simulink model "gmStateSpaceHDL_uz_inverter_3ph"  (R2021b)
settings: Solver=FixedStepDiscrete  StartTime=0.0  StopTime=0.1  FixedStep=Auto  RelTol=1e-3
InitFcn:
  | load('C:\Users\valen\Documents\repos\2021_10_hoppe_hoerner_regelung_neunstraengige_pmsm\sschdl\uz_inverter_3ph\stateSpaceParameters.mat');
values from neighbouring files (symbols this model uses):
  udc = 200    [uz_inverter_3ph_init_parameter.m]
undefined symbols (not defined in the file or in its folder): stateSpaceParameters_1
libraries: simulink x17, hdlsllib x2, hdlssclib x2
settings Model: Creator=LENOVO  LastModifiedBy=valen
settings SolverCC: AlgebraicLoopSolver=TrustRegion
settings DataIOCC: LimitDataPoints=on  SaveOutput=off  SaveTime=off
settings OptimizationCC: BlockReduction=off  ConditionallyExecuteInputs=off  DefaultParameterBehavior=Inlined  InheritOutputTypeSmallerThanSingle=on  LifeSpan=inf
settings DebuggingCC: AlgebraicLoopMsg=error  SingleTaskRateTransMsg=error  AllowSymbolicDim=off  StrictBusMsg=ErrorOnBusTreatedAsVector  SFUnexpectedBacktrackingDiag=warning  SFNoUnconditionalDefaultTransitionDiag=warning  SFExecutionAtInitializationDiag=none  SFMachineParentedDataDiag=warning  ArithmeticOperatorsInVariantConditions=warning
settings HardwareCC: ProdBitPerPointer=32  ProdBitPerSizeT=32  ProdBitPerPtrDiffT=32  ProdLargestAtomicFloat=None  ProdIntDivRoundTo=Undefined  ProdEndianess=Unspecified  ProdWordSize=32  ProdHWDeviceType=ASIC/FPGA->ASIC/FPGA  ProdEqTarget=off
settings SFSimCC: SimUseLocalCustomCode=off  CustomCodeUndefinedFunction=UseInterfaceOnly
settings RTWCC: RTWUseLocalCustomCode=off
settings CodeAppCC: StateflowObjectComments=on
settings GRTTargetCC: TargetLangStandard=C89/C90 (ANSI)
settings ConfigComp: CovScope=ReferencedModels  CovMetricSettings=dw  CovSaveCumulativeToWorkspaceVar=on  CovSaveSingleToWorkspaceVar=on  CovExternalEMLEnable=off  CovSFcnEnable=off

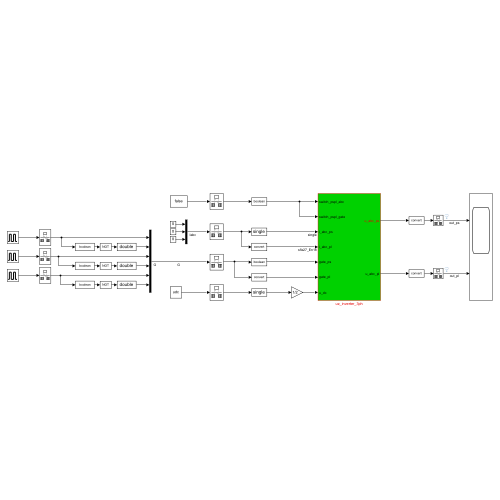
[thumbnail: Simulink's stored preview of the top-level diagram]
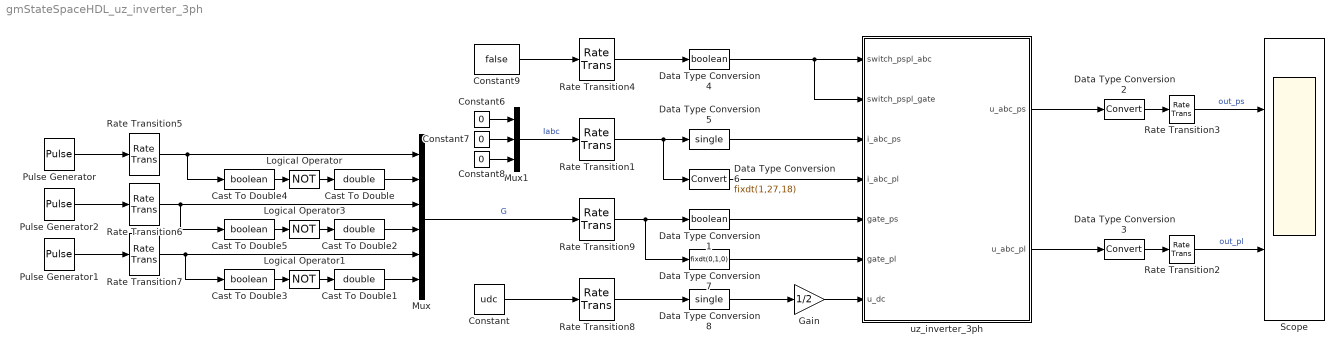
== system gmStateSpaceHDL_uz_inverter_3ph ==
  Cast To Double : DataTypeConversion  OutDataTypeStr=double
  Cast To Double1 : DataTypeConversion  OutDataTypeStr=double
  Cast To Double2 : DataTypeConversion  OutDataTypeStr=double
  Cast To Double3 : DataTypeConversion  OutDataTypeStr=boolean
  Cast To Double4 : DataTypeConversion  OutDataTypeStr=boolean
  Cast To Double5 : DataTypeConversion  OutDataTypeStr=boolean
  Constant : Constant  Value=udc
  Constant6 : Constant  Value=0
  Constant7 : Constant  Value=0
  Constant8 : Constant  Value=0
  Constant9 : Constant  Value=false
  Data Type Conversion1 : DataTypeConversion  OutDataTypeStr=boolean  RndMeth=Nearest
  Data Type Conversion2 : DataTypeConversion
  Data Type Conversion3 : DataTypeConversion
  Data Type Conversion4 : DataTypeConversion  OutDataTypeStr=boolean
  Data Type Conversion5 : DataTypeConversion  OutDataTypeStr=single  RndMeth=Nearest
  Data Type Conversion6 : DataTypeConversion  OutDataTypeStr=fixdt(1,27,18)  RndMeth=Nearest
  Data Type Conversion7 : DataTypeConversion  OutDataTypeStr=fixdt(0,1,0)  RndMeth=Nearest
  Data Type Conversion8 : DataTypeConversion  OutDataTypeStr=single  RndMeth=Nearest
  Gain : Gain  Gain=1/2  OutDataTypeStr=Inherit: Same as input
  Logical Operator : Logic  Operator=NOT  AllPortsSameDT=off  OutDataTypeStr=boolean
  Logical Operator1 : Logic  Operator=NOT  AllPortsSameDT=off  OutDataTypeStr=boolean
  Logical Operator3 : Logic  Operator=NOT  AllPortsSameDT=off  OutDataTypeStr=boolean
  Mux : Mux  Inputs=6
  Mux1 : Mux  Inputs=3
  Pulse Generator : DiscretePulseGenerator  PulseType=Time based  Period=0.001  PulseWidth=50
  Pulse Generator1 : DiscretePulseGenerator  PulseType=Time based  Period=0.01  PulseWidth=50
  Pulse Generator2 : DiscretePulseGenerator  PulseType=Time based  Period=0.05  PulseWidth=50
  Rate Transition{1..9} (9 alike) : RateTransition  OutPortSampleTime=ts_inverter
  Scope : Scope  NumInputPorts=2
  uz_inverter_3ph : Subsystem
  wires:
  uz_inverter_3ph/1(u_abc_ps) -> Data Type Conversion2/1
  uz_inverter_3ph/2(u_abc_pl) -> Data Type Conversion3/1
  Data Type Conversion3/1 -> Rate Transition2/1
  Data Type Conversion2/1 -> Rate Transition3/1
  Rate Transition3/1 -> Scope/1  "out_ps"
  Rate Transition2/1 -> Scope/2  "out_pl"
  Constant9/1 -> Rate Transition4/1
  Rate Transition4/1 -> Data Type Conversion4/1
  Mux1/1 -> Rate Transition1/1  "Iabc"
  Constant8/1 -> Mux1/3
  Constant6/1 -> Mux1/1
  Constant7/1 -> Mux1/2
  Rate Transition1/1 -> Data Type Conversion5/1, Data Type Conversion6/1
  Data Type Conversion6/1 -> uz_inverter_3ph/4(i_abc_pl)
  Rate Transition9/1 -> Data Type Conversion7/1, Data Type Conversion1/1
  Data Type Conversion1/1 -> uz_inverter_3ph/5(gate_ps)
  Data Type Conversion5/1 -> uz_inverter_3ph/3(i_abc_ps)
  Data Type Conversion7/1 -> uz_inverter_3ph/6(gate_pl)
  Logical Operator1/1 -> Cast To Double1/1
  Cast To Double3/1 -> Logical Operator1/1
  Pulse Generator1/1 -> Rate Transition7/1
  Cast To Double5/1 -> Logical Operator3/1
  Logical Operator3/1 -> Cast To Double2/1
  Pulse Generator2/1 -> Rate Transition6/1
  Pulse Generator/1 -> Rate Transition5/1
  Cast To Double2/1 -> Mux/4
  Cast To Double4/1 -> Logical Operator/1
  Cast To Double1/1 -> Mux/6
  Logical Operator/1 -> Cast To Double/1
  Mux/1 -> Rate Transition9/1  "G"
  Cast To Double/1 -> Mux/2
  Rate Transition7/1 -> Cast To Double3/1, Mux/5
  Data Type Conversion8/1 -> Gain/1
  Constant/1 -> Rate Transition8/1
  Rate Transition8/1 -> Data Type Conversion8/1
  Gain/1 -> uz_inverter_3ph/7(u_dc)
  Rate Transition6/1 -> Cast To Double5/1, Mux/3
  Rate Transition5/1 -> Cast To Double4/1, Mux/1
  Data Type Conversion4/1 -> uz_inverter_3ph/2(switch_pspl_gate), uz_inverter_3ph/1(switch_pspl_abc)

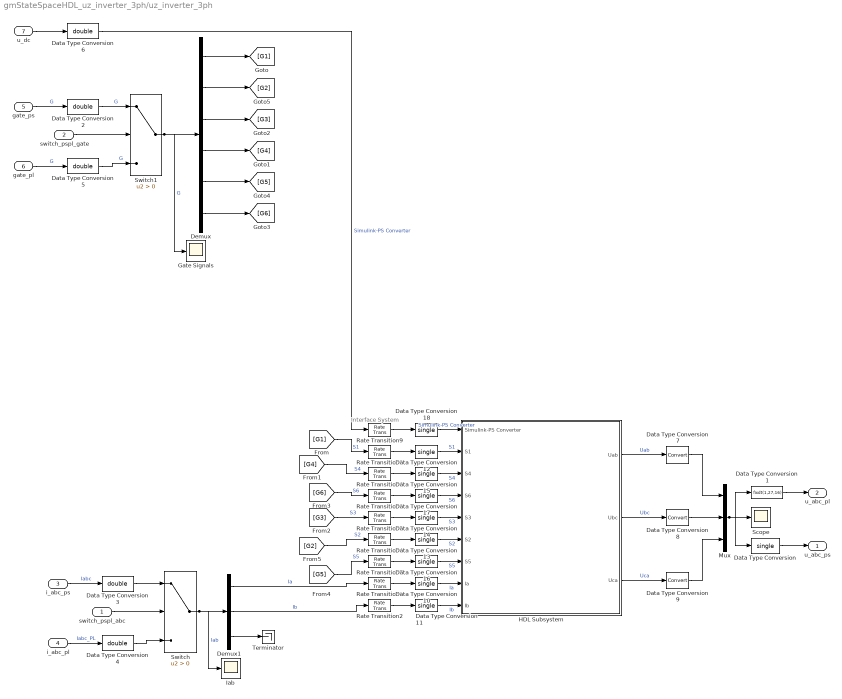
== system gmStateSpaceHDL_uz_inverter_3ph/uz_inverter_3ph ==
  note: Interface System
  switch_pspl_abc : Inport
  switch_pspl_gate : Inport  Port=2
  i_abc_ps : Inport  Port=3  OutDataTypeStr=single
  i_abc_pl : Inport  Port=4  OutDataTypeStr=fixdt(1,27,18)
  gate_ps : Inport  Port=5  LockScale=on
  gate_pl : Inport  Port=6  LockScale=on
  u_dc : Inport  Port=7
  Data Type Conversion{,10..18} (10 alike) : DataTypeConversion  OutDataTypeStr=single  RndMeth=Nearest
  Data Type Conversion1 : DataTypeConversion  OutDataTypeStr=fixdt(1,27,16)  RndMeth=Nearest
  Data Type Conversion{2..6} (5 alike) : DataTypeConversion  OutDataTypeStr=double  RndMeth=Nearest
  Data Type Conversion7 : DataTypeConversion  RndMeth=Nearest
  Data Type Conversion8 : DataTypeConversion  RndMeth=Nearest
  Data Type Conversion9 : DataTypeConversion  RndMeth=Nearest
  Demux : Demux  Outputs=6
  Demux1 : Demux  Outputs=3
  Gate Signals : Scope
  HDL Subsystem : Subsystem
  Iab : Scope
  Mux : Mux  Inputs=3
  Rate Transition{1..9} (9 alike) : RateTransition  OutPortSampleTime=1e-06
  Scope : Scope
  Switch : Switch  Criteria=u2 > Threshold
  Switch1 : Switch  Criteria=u2 > Threshold
  Terminator : Terminator
  u_abc_ps : Outport
  u_abc_pl : Outport  Port=2
  wires:
  Data Type Conversion17/1 -> HDL Subsystem/4(S6)  "S6"
  Rate Transition3/1 -> Data Type Conversion12/1
  Data Type Conversion16/1 -> HDL Subsystem/7(S5)  "S5"
  Mux/1 -> Data Type Conversion/1, Scope/1, Data Type Conversion1/1
  Rate Transition9/1 -> Data Type Conversion18/1
  Data Type Conversion10/1 -> HDL Subsystem/8(Ia)  "Ia"
  Data Type Conversion11/1 -> HDL Subsystem/9(Ib)  "Ib"
  Data Type Conversion5/1 -> Switch1/3  "G"
  Switch/1 -> Demux1/1, Iab/1  "Iab"
  i_abc_pl/1 -> Data Type Conversion4/1  "Iabc_PL"
  Data Type Conversion14/1 -> HDL Subsystem/5(S3)  "S3"
  Demux/1 -> [G1]
  Data Type Conversion4/1 -> Switch/3
  Data Type Conversion3/1 -> Switch/1
  Data Type Conversion13/1 -> HDL Subsystem/6(S2)  "S2"
  gate_pl/1 -> Data Type Conversion5/1  "G"
  switch_pspl_abc/1 -> Switch/2
  Data Type Conversion15/1 -> HDL Subsystem/3(S4)  "S4"
  Rate Transition4/1 -> Data Type Conversion13/1
  Data Type Conversion12/1 -> HDL Subsystem/2(S1)  "S1"
  Data Type Conversion18/1 -> HDL Subsystem/1(Simulink-PS Converter)  "Simulink-PS Converter"
  Rate Transition8/1 -> Data Type Conversion17/1
  Rate Transition7/1 -> Data Type Conversion16/1
  Demux/3 -> [G3]
  Rate Transition6/1 -> Data Type Conversion15/1
  Demux/4 -> [G4]
  Rate Transition5/1 -> Data Type Conversion14/1
  Data Type Conversion/1 -> u_abc_ps/1
  Rate Transition2/1 -> Data Type Conversion11/1
  Rate Transition1/1 -> Data Type Conversion10/1
  Data Type Conversion1/1 -> u_abc_pl/1
  Demux/2 -> [G2]
  Demux1/3 -> Terminator/1
  i_abc_ps/1 -> Data Type Conversion3/1  "Iabc"
  gate_ps/1 -> Data Type Conversion2/1  "G"
  Demux/6 -> [G6]
  u_dc/1 -> Data Type Conversion6/1
  Data Type Conversion2/1 -> Switch1/1  "G"
  Switch1/1 -> Demux/1, Gate Signals/1  "G"
  switch_pspl_gate/1 -> Switch1/2
  Demux/5 -> [G5]
  [G1] -> Rate Transition3/1  "S1"
  Data Type Conversion7/1 -> Mux/1
  [G2] -> Rate Transition4/1  "S2"
  Data Type Conversion9/1 -> Mux/3
  [G3] -> Rate Transition5/1  "S3"
  Data Type Conversion8/1 -> Mux/2
  [G4] -> Rate Transition6/1  "S4"
  [G5] -> Rate Transition7/1  "S5"
  [G6] -> Rate Transition8/1  "S6"
  HDL Subsystem/1(Uab) -> Data Type Conversion7/1  "Uab"
  HDL Subsystem/2(Ubc) -> Data Type Conversion8/1  "Ubc"
  HDL Subsystem/3(Uca) -> Data Type Conversion9/1  "Uca"
  Demux1/1 -> Rate Transition1/1  "Ia"
  Demux1/2 -> Rate Transition2/1  "Ib"
  Data Type Conversion6/1 -> Rate Transition9/1  "Simulink-PS Converter"

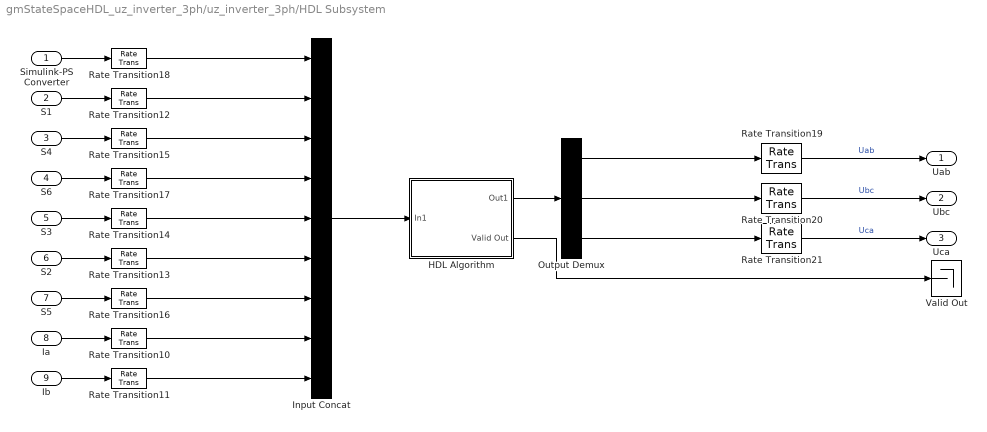
== system gmStateSpaceHDL_uz_inverter_3ph/uz_inverter_3ph/HDL Subsystem ==
  Simulink-PS Converter : Inport
  S1 : Inport  Port=2
  S4 : Inport  Port=3
  S6 : Inport  Port=4
  S3 : Inport  Port=5
  S2 : Inport  Port=6
  S5 : Inport  Port=7
  Ia : Inport  Port=8
  Ib : Inport  Port=9
  HDL Algorithm : Subsystem
  Input Concat : Concatenate  NumInputs=9
  Output Demux : Demux  Outputs=3
  Rate Transition{10..18} (9 alike) : RateTransition  Integrity=off  OutPortSampleTimeOpt=Multiple of input port sample time  OutPortSampleTimeMultiple=1/4
  Rate Transition19 : RateTransition  OutPortSampleTimeOpt=Multiple of input port sample time  OutPortSampleTimeMultiple=4
  Rate Transition20 : RateTransition  OutPortSampleTimeOpt=Multiple of input port sample time  OutPortSampleTimeMultiple=4
  Rate Transition21 : RateTransition  OutPortSampleTimeOpt=Multiple of input port sample time  OutPortSampleTimeMultiple=4
  Valid Out : Terminator
  Uab : Outport
  Ubc : Outport  Port=2
  Uca : Outport  Port=3
  wires:
  Rate Transition12/1 -> Input Concat/2
  Rate Transition13/1 -> Input Concat/6
  Output Demux/1 -> Rate Transition19/1
  Rate Transition14/1 -> Input Concat/5
  Rate Transition18/1 -> Input Concat/1
  Ib/1 -> Rate Transition11/1
  Rate Transition17/1 -> Input Concat/4
  HDL Algorithm/2(Valid Out) -> Valid Out/1
  Input Concat/1 -> HDL Algorithm/1(In1)
  HDL Algorithm/1(Out1) -> Output Demux/1
  Rate Transition15/1 -> Input Concat/3
  S1/1 -> Rate Transition12/1
  Output Demux/3 -> Rate Transition21/1
  Rate Transition11/1 -> Input Concat/9
  Output Demux/2 -> Rate Transition20/1
  S2/1 -> Rate Transition13/1
  Rate Transition16/1 -> Input Concat/7
  Rate Transition10/1 -> Input Concat/8
  Rate Transition19/1 -> Uab/1  "Uab"
  S4/1 -> Rate Transition15/1
  S6/1 -> Rate Transition17/1
  Simulink-PS Converter/1 -> Rate Transition18/1
  Rate Transition21/1 -> Uca/1  "Uca"
  Ia/1 -> Rate Transition10/1
  S5/1 -> Rate Transition16/1
  Rate Transition20/1 -> Ubc/1  "Ubc"
  S3/1 -> Rate Transition14/1

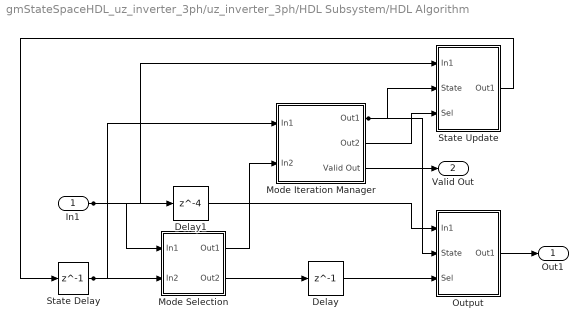
== system gmStateSpaceHDL_uz_inverter_3ph/uz_inverter_3ph/HDL Subsystem/HDL Algorithm ==
  In1 : Inport
  Delay : Delay  DelayLength=1
  Delay1 : Delay  DelayLength=4
  Mode Iteration Manager : Subsystem
  Mode Selection : Subsystem
  Output : Subsystem
  State Delay : Delay  DelayLength=1  InitialCondition=single(stateSpaceParameters_1.X0)
  State Update : Subsystem
  Out1 : Outport  VectorParamsAs1DForOutWhenUnconnected=off
  Valid Out : Outport  Port=2  VectorParamsAs1DForOutWhenUnconnected=off
  wires:
  Mode Iteration Manager/3(Valid Out) -> Valid Out/1
  Output/1(Out1) -> Out1/1
  Mode Selection/1(Out1) -> Mode Iteration Manager/2(In2)
  State Update/1(Out1) -> State Delay/1
  Delay1/1 -> Output/1(In1)
  Mode Selection/2(Out2) -> Delay/1
  Mode Iteration Manager/2(Out2) -> State Update/3(Sel)
  Delay/1 -> Output/3(Sel)
  State Delay/1 -> Mode Selection/2(In2), Mode Iteration Manager/1(In1)
  Mode Iteration Manager/1(Out1) -> Output/2(State), State Update/2(State)
  In1/1 -> Mode Selection/1(In1), State Update/1(In1), Delay1/1

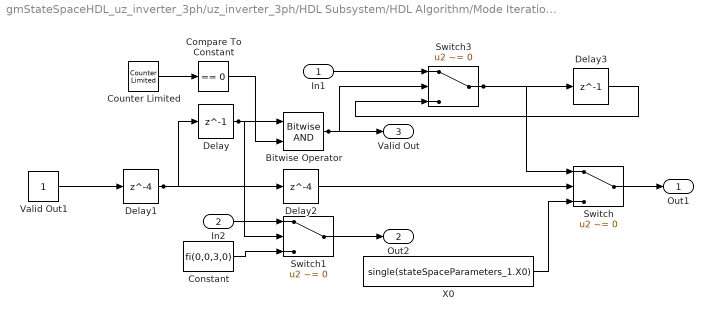
== system gmStateSpaceHDL_uz_inverter_3ph/uz_inverter_3ph/HDL Subsystem/HDL Algorithm/Mode Iteration Manager ==
  In1 : Inport
  In2 : Inport  Port=2
  Bitwise Operator : simulink/Logic and Bit Operations/Bitwise Operator  logicop=AND  UseBitMask=off  NumInputPorts=2  BitMask=bin2dec('11011001')  BitMaskRealWorld=Stored Integer
  Compare To Constant : hdlsllib/Logic and Bit Operations/Compare To Constant  relop===  const=0  OutDataTypeStr=boolean
      settings: SourceProductBaseCode=SL
  Constant : Constant  Value=fi(0,0,3,0)  SampleTime=2.5e-07
  Counter Limited : hdlsllib/Sources/Counter Limited  uplimit=3  tsamp=-1
      settings: SourceProductBaseCode=SL
  Delay : Delay  DelayLength=1
  Delay1 : Delay  DelayLength=4
  Delay2 : Delay  DelayLength=4
  Delay3 : Delay  DelayLength=1
  Switch : Switch  Criteria=u2 ~= 0
  Switch1 : Switch  Criteria=u2 ~= 0
  Switch3 : Switch  Criteria=u2 ~= 0
  Valid Out1 : Constant  OutDataTypeStr=boolean  SampleTime=2.5e-07
  X0 : Constant  Value=single(stateSpaceParameters_1.X0)  SampleTime=2.5e-07
  Out1 : Outport  OutDataTypeStr=single  VectorParamsAs1DForOutWhenUnconnected=off
  Out2 : Outport  Port=2  VectorParamsAs1DForOutWhenUnconnected=off
  Valid Out : Outport  Port=3  VectorParamsAs1DForOutWhenUnconnected=off
  wires:
  Counter Limited/1 -> Compare To Constant/1
  In1/1 -> Switch3/1
  Delay3/1 -> Switch3/3
  Compare To Constant/1 -> Bitwise Operator/2
  Switch/1 -> Out1/1
  In2/1 -> Switch1/1
  Switch1/1 -> Out2/1
  Constant/1 -> Switch1/3
  X0/1 -> Switch/3
  Delay2/1 -> Switch/2
  Valid Out1/1 -> Delay1/1
  Switch3/1 -> Delay3/1, Switch/1
  Delay/1 -> Switch1/2, Bitwise Operator/1
  Bitwise Operator/1 -> Valid Out/1, Switch3/2
  Delay1/1 -> Delay2/1, Delay/1

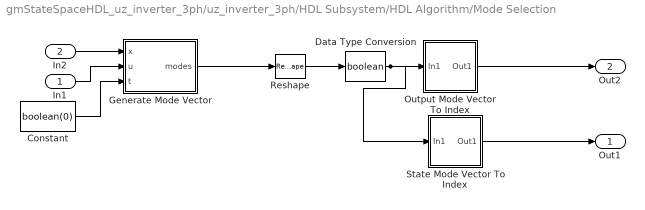
== system gmStateSpaceHDL_uz_inverter_3ph/uz_inverter_3ph/HDL Subsystem/HDL Algorithm/Mode Selection ==
  In1 : Inport
  In2 : Inport  Port=2
  Constant : Constant  Value=boolean(0)  SampleTime=2.5e-07
  Data Type Conversion : DataTypeConversion  OutDataTypeStr=boolean
  Generate Mode Vector : MATLAB Function  TreatAsAtomicUnit=on
  Output Mode Vector To Index : Subsystem
  Reshape : Reshape
  State Mode Vector To Index : Subsystem
  Out1 : Outport  VectorParamsAs1DForOutWhenUnconnected=off
  Out2 : Outport  Port=2  VectorParamsAs1DForOutWhenUnconnected=off
  wires:
  Output Mode Vector To Index/1(Out1) -> Out2/1
  Constant/1 -> Generate Mode Vector/3(t)
  State Mode Vector To Index/1(Out1) -> Out1/1
  In1/1 -> Generate Mode Vector/2(u)
  Reshape/1 -> Data Type Conversion/1
  Generate Mode Vector/1(modes) -> Reshape/1
  In2/1 -> Generate Mode Vector/1(x)
  Data Type Conversion/1 -> State Mode Vector To Index/1(In1), Output Mode Vector To Index/1(In1)

== system gmStateSpaceHDL_uz_inverter_3ph/uz_inverter_3ph/HDL Subsystem/HDL Algorithm/Output ==
  In1 : Inport
  State : Inport  Port=2
  Sel : Inport  Port=3
  Bias : Terminator
  Multiply Input : Terminator
  Multiply State : hdlssclib/NFPSparseConstMultiply  constMatrix=single(stateSpaceParameters_1.Cd)
      settings: SourceProductBaseCode=SL
  Out1 : Outport  VectorParamsAs1DForOutWhenUnconnected=off
  wires:
  State/1 -> Multiply State/1
  In1/1 -> Multiply Input/1
  Sel/1 -> Bias/1, Multiply State/2
  Multiply State/1 -> Out1/1

== system gmStateSpaceHDL_uz_inverter_3ph/uz_inverter_3ph/HDL Subsystem/HDL Algorithm/State Update ==
  In1 : Inport
  State : Inport  Port=2
  Sel : Inport  Port=3
  Bias : Terminator
  Multiply Input : hdlssclib/NFPSparseConstMultiply  constMatrix=single(stateSpaceParameters_1.Bd)
      settings: SourceProductBaseCode=SL
  Multiply State : Terminator
  Out1 : Outport  OutDataTypeStr=single  VectorParamsAs1DForOutWhenUnconnected=off
  wires:
  State/1 -> Multiply State/1
  In1/1 -> Multiply Input/1
  Sel/1 -> Bias/1, Multiply Input/2
  Multiply Input/1 -> Out1/1

== system gmStateSpaceHDL_uz_inverter_3ph/uz_inverter_3ph/HDL Subsystem/HDL Algorithm/Mode Selection/Output Mode Vector To Index ==
  In1 : Inport
  Index : Constant  Value=fi(0,0,1,0)  SampleTime=2.5e-07
  Term : Terminator
  Out1 : Outport  VectorParamsAs1DForOutWhenUnconnected=off
  wires:
  In1/1 -> Term/1
  Index/1 -> Out1/1

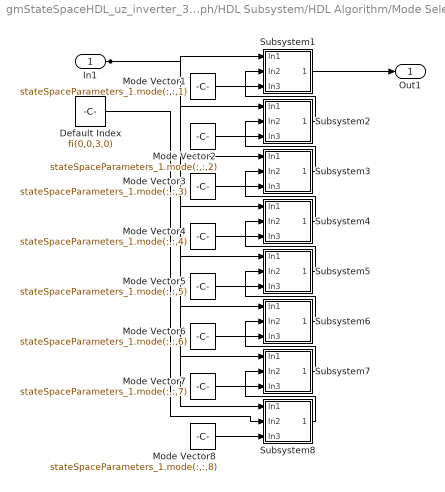
== system gmStateSpaceHDL_uz_inverter_3ph/uz_inverter_3ph/HDL Subsystem/HDL Algorithm/Mode Selection/State Mode Vector To Index ==
  In1 : Inport
  Default Index : Constant  Value=fi(0,0,3,0)  SampleTime=2.5e-07
  Mode Vector1 : Constant  Value=stateSpaceParameters_1.mode(:,:,1)  OutDataTypeStr=boolean  SampleTime=2.5e-07
  Mode Vector2 : Constant  Value=stateSpaceParameters_1.mode(:,:,2)  OutDataTypeStr=boolean  SampleTime=2.5e-07
  Mode Vector3 : Constant  Value=stateSpaceParameters_1.mode(:,:,3)  OutDataTypeStr=boolean  SampleTime=2.5e-07
  Mode Vector4 : Constant  Value=stateSpaceParameters_1.mode(:,:,4)  OutDataTypeStr=boolean  SampleTime=2.5e-07
  Mode Vector5 : Constant  Value=stateSpaceParameters_1.mode(:,:,5)  OutDataTypeStr=boolean  SampleTime=2.5e-07
  Mode Vector6 : Constant  Value=stateSpaceParameters_1.mode(:,:,6)  OutDataTypeStr=boolean  SampleTime=2.5e-07
  Mode Vector7 : Constant  Value=stateSpaceParameters_1.mode(:,:,7)  OutDataTypeStr=boolean  SampleTime=2.5e-07
  Mode Vector8 : Constant  Value=stateSpaceParameters_1.mode(:,:,8)  OutDataTypeStr=boolean  SampleTime=2.5e-07
  Subsystem1 : Subsystem  TreatAsAtomicUnit=on  mask{Index=fi(0,0,3,0)}
  Subsystem2 : Subsystem  TreatAsAtomicUnit=on  mask{Index=fi(1,0,3,0)}
  Subsystem3 : Subsystem  TreatAsAtomicUnit=on  mask{Index=fi(2,0,3,0)}
  Subsystem4 : Subsystem  TreatAsAtomicUnit=on  mask{Index=fi(3,0,3,0)}
  Subsystem5 : Subsystem  TreatAsAtomicUnit=on  mask{Index=fi(4,0,3,0)}
  Subsystem6 : Subsystem  TreatAsAtomicUnit=on  mask{Index=fi(5,0,3,0)}
  Subsystem7 : Subsystem  TreatAsAtomicUnit=on  mask{Index=fi(6,0,3,0)}
  Subsystem8 : Subsystem  TreatAsAtomicUnit=on  mask{Index=fi(7,0,3,0)}
  Out1 : Outport  VectorParamsAs1DForOutWhenUnconnected=off
  wires:
  Mode Vector1/1 -> Subsystem1/3(In3)
  Mode Vector2/1 -> Subsystem2/3(In3)
  Mode Vector3/1 -> Subsystem3/3(In3)
  Mode Vector4/1 -> Subsystem4/3(In3)
  Mode Vector5/1 -> Subsystem5/3(In3)
  Mode Vector6/1 -> Subsystem6/3(In3)
  Mode Vector7/1 -> Subsystem7/3(In3)
  Mode Vector8/1 -> Subsystem8/3(In3)
  In1/1 -> Subsystem1/1(In1), Subsystem2/1(In1), Subsystem3/1(In1), Subsystem4/1(In1), Subsystem5/1(In1), Subsystem6/1(In1), Subsystem7/1(In1), Subsystem8/1(In1)
  Subsystem2/1(Out1) -> Subsystem1/2(In2)
  Subsystem3/1(Out1) -> Subsystem2/2(In2)
  Subsystem4/1(Out1) -> Subsystem3/2(In2)
  Subsystem5/1(Out1) -> Subsystem4/2(In2)
  Subsystem6/1(Out1) -> Subsystem5/2(In2)
  Subsystem7/1(Out1) -> Subsystem6/2(In2)
  Subsystem8/1(Out1) -> Subsystem7/2(In2)
  Subsystem1/1(Out1) -> Out1/1
  Default Index/1 -> Subsystem8/2(In2)

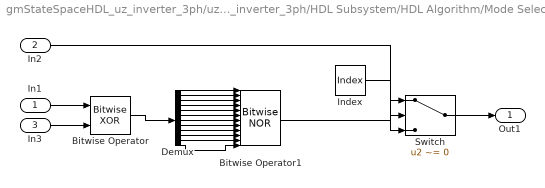
== system gmStateSpaceHDL_uz_inverter_3ph/uz_inverter_3ph/HDL Subsystem/HDL Algorithm/Mode Selection/State Mode Vector To Index/Subsystem1 ==
  In1 : Inport
  In2 : Inport  Port=2
  In3 : Inport  Port=3
  Bitwise Operator : simulink/Logic and Bit Operations/Bitwise Operator  logicop=XOR  UseBitMask=off  NumInputPorts=2  BitMask=bin2dec('11011001')  BitMaskRealWorld=Stored Integer
  Bitwise Operator1 : simulink/Logic and Bit Operations/Bitwise Operator  logicop=NOR  UseBitMask=off  NumInputPorts=12  BitMask=bin2dec('11011001')  BitMaskRealWorld=Stored Integer
  Demux : Demux  Outputs=12
  Index : Constant  Value=Index  SampleTime=2.5e-07
  Switch : Switch  Criteria=u2 ~= 0
  Out1 : Outport  VectorParamsAs1DForOutWhenUnconnected=off
  wires:
  In1/1 -> Bitwise Operator/1
  In3/1 -> Bitwise Operator/2
  Bitwise Operator/1 -> Demux/1
  Demux/1 -> Bitwise Operator1/1
  Demux/2 -> Bitwise Operator1/2
  Demux/3 -> Bitwise Operator1/3
  Demux/4 -> Bitwise Operator1/4
  Demux/5 -> Bitwise Operator1/5
  Demux/6 -> Bitwise Operator1/6
  Demux/7 -> Bitwise Operator1/7
  Demux/8 -> Bitwise Operator1/8
  Demux/9 -> Bitwise Operator1/9
  Demux/10 -> Bitwise Operator1/10
  Demux/11 -> Bitwise Operator1/11
  Demux/12 -> Bitwise Operator1/12
  In2/1 -> Switch/3
  Bitwise Operator1/1 -> Switch/2
  Switch/1 -> Out1/1
  Index/1 -> Switch/1

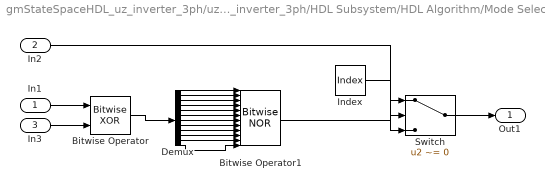
== system gmStateSpaceHDL_uz_inverter_3ph/uz_inverter_3ph/HDL Subsystem/HDL Algorithm/Mode Selection/State Mode Vector To Index/Subsystem2 ==
  In1 : Inport
  In2 : Inport  Port=2
  In3 : Inport  Port=3
  Bitwise Operator : simulink/Logic and Bit Operations/Bitwise Operator  logicop=XOR  UseBitMask=off  NumInputPorts=2  BitMask=bin2dec('11011001')  BitMaskRealWorld=Stored Integer
  Bitwise Operator1 : simulink/Logic and Bit Operations/Bitwise Operator  logicop=NOR  UseBitMask=off  NumInputPorts=12  BitMask=bin2dec('11011001')  BitMaskRealWorld=Stored Integer
  Demux : Demux  Outputs=12
  Index : Constant  Value=Index  SampleTime=2.5e-07
  Switch : Switch  Criteria=u2 ~= 0
  Out1 : Outport  VectorParamsAs1DForOutWhenUnconnected=off
  wires:
  In1/1 -> Bitwise Operator/1
  In3/1 -> Bitwise Operator/2
  Bitwise Operator/1 -> Demux/1
  Demux/1 -> Bitwise Operator1/1
  Demux/2 -> Bitwise Operator1/2
  Demux/3 -> Bitwise Operator1/3
  Demux/4 -> Bitwise Operator1/4
  Demux/5 -> Bitwise Operator1/5
  Demux/6 -> Bitwise Operator1/6
  Demux/7 -> Bitwise Operator1/7
  Demux/8 -> Bitwise Operator1/8
  Demux/9 -> Bitwise Operator1/9
  Demux/10 -> Bitwise Operator1/10
  Demux/11 -> Bitwise Operator1/11
  Demux/12 -> Bitwise Operator1/12
  In2/1 -> Switch/3
  Bitwise Operator1/1 -> Switch/2
  Switch/1 -> Out1/1
  Index/1 -> Switch/1

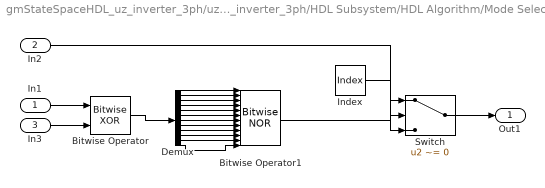
== system gmStateSpaceHDL_uz_inverter_3ph/uz_inverter_3ph/HDL Subsystem/HDL Algorithm/Mode Selection/State Mode Vector To Index/Subsystem3 ==
  In1 : Inport
  In2 : Inport  Port=2
  In3 : Inport  Port=3
  Bitwise Operator : simulink/Logic and Bit Operations/Bitwise Operator  logicop=XOR  UseBitMask=off  NumInputPorts=2  BitMask=bin2dec('11011001')  BitMaskRealWorld=Stored Integer
  Bitwise Operator1 : simulink/Logic and Bit Operations/Bitwise Operator  logicop=NOR  UseBitMask=off  NumInputPorts=12  BitMask=bin2dec('11011001')  BitMaskRealWorld=Stored Integer
  Demux : Demux  Outputs=12
  Index : Constant  Value=Index  SampleTime=2.5e-07
  Switch : Switch  Criteria=u2 ~= 0
  Out1 : Outport  VectorParamsAs1DForOutWhenUnconnected=off
  wires:
  In1/1 -> Bitwise Operator/1
  In3/1 -> Bitwise Operator/2
  Bitwise Operator/1 -> Demux/1
  Demux/1 -> Bitwise Operator1/1
  Demux/2 -> Bitwise Operator1/2
  Demux/3 -> Bitwise Operator1/3
  Demux/4 -> Bitwise Operator1/4
  Demux/5 -> Bitwise Operator1/5
  Demux/6 -> Bitwise Operator1/6
  Demux/7 -> Bitwise Operator1/7
  Demux/8 -> Bitwise Operator1/8
  Demux/9 -> Bitwise Operator1/9
  Demux/10 -> Bitwise Operator1/10
  Demux/11 -> Bitwise Operator1/11
  Demux/12 -> Bitwise Operator1/12
  In2/1 -> Switch/3
  Bitwise Operator1/1 -> Switch/2
  Switch/1 -> Out1/1
  Index/1 -> Switch/1

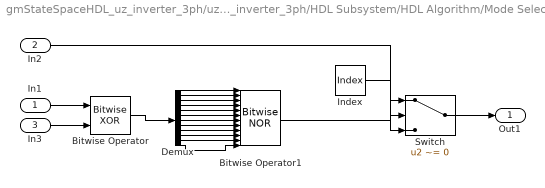
== system gmStateSpaceHDL_uz_inverter_3ph/uz_inverter_3ph/HDL Subsystem/HDL Algorithm/Mode Selection/State Mode Vector To Index/Subsystem4 ==
  In1 : Inport
  In2 : Inport  Port=2
  In3 : Inport  Port=3
  Bitwise Operator : simulink/Logic and Bit Operations/Bitwise Operator  logicop=XOR  UseBitMask=off  NumInputPorts=2  BitMask=bin2dec('11011001')  BitMaskRealWorld=Stored Integer
  Bitwise Operator1 : simulink/Logic and Bit Operations/Bitwise Operator  logicop=NOR  UseBitMask=off  NumInputPorts=12  BitMask=bin2dec('11011001')  BitMaskRealWorld=Stored Integer
  Demux : Demux  Outputs=12
  Index : Constant  Value=Index  SampleTime=2.5e-07
  Switch : Switch  Criteria=u2 ~= 0
  Out1 : Outport  VectorParamsAs1DForOutWhenUnconnected=off
  wires:
  In1/1 -> Bitwise Operator/1
  In3/1 -> Bitwise Operator/2
  Bitwise Operator/1 -> Demux/1
  Demux/1 -> Bitwise Operator1/1
  Demux/2 -> Bitwise Operator1/2
  Demux/3 -> Bitwise Operator1/3
  Demux/4 -> Bitwise Operator1/4
  Demux/5 -> Bitwise Operator1/5
  Demux/6 -> Bitwise Operator1/6
  Demux/7 -> Bitwise Operator1/7
  Demux/8 -> Bitwise Operator1/8
  Demux/9 -> Bitwise Operator1/9
  Demux/10 -> Bitwise Operator1/10
  Demux/11 -> Bitwise Operator1/11
  Demux/12 -> Bitwise Operator1/12
  In2/1 -> Switch/3
  Bitwise Operator1/1 -> Switch/2
  Switch/1 -> Out1/1
  Index/1 -> Switch/1

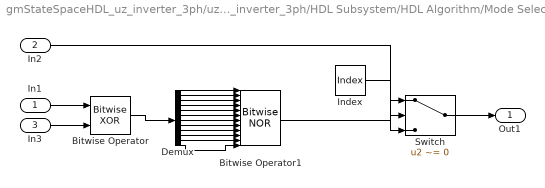
== system gmStateSpaceHDL_uz_inverter_3ph/uz_inverter_3ph/HDL Subsystem/HDL Algorithm/Mode Selection/State Mode Vector To Index/Subsystem5 ==
  In1 : Inport
  In2 : Inport  Port=2
  In3 : Inport  Port=3
  Bitwise Operator : simulink/Logic and Bit Operations/Bitwise Operator  logicop=XOR  UseBitMask=off  NumInputPorts=2  BitMask=bin2dec('11011001')  BitMaskRealWorld=Stored Integer
  Bitwise Operator1 : simulink/Logic and Bit Operations/Bitwise Operator  logicop=NOR  UseBitMask=off  NumInputPorts=12  BitMask=bin2dec('11011001')  BitMaskRealWorld=Stored Integer
  Demux : Demux  Outputs=12
  Index : Constant  Value=Index  SampleTime=2.5e-07
  Switch : Switch  Criteria=u2 ~= 0
  Out1 : Outport  VectorParamsAs1DForOutWhenUnconnected=off
  wires:
  In1/1 -> Bitwise Operator/1
  In3/1 -> Bitwise Operator/2
  Bitwise Operator/1 -> Demux/1
  Demux/1 -> Bitwise Operator1/1
  Demux/2 -> Bitwise Operator1/2
  Demux/3 -> Bitwise Operator1/3
  Demux/4 -> Bitwise Operator1/4
  Demux/5 -> Bitwise Operator1/5
  Demux/6 -> Bitwise Operator1/6
  Demux/7 -> Bitwise Operator1/7
  Demux/8 -> Bitwise Operator1/8
  Demux/9 -> Bitwise Operator1/9
  Demux/10 -> Bitwise Operator1/10
  Demux/11 -> Bitwise Operator1/11
  Demux/12 -> Bitwise Operator1/12
  In2/1 -> Switch/3
  Bitwise Operator1/1 -> Switch/2
  Switch/1 -> Out1/1
  Index/1 -> Switch/1

== system gmStateSpaceHDL_uz_inverter_3ph/uz_inverter_3ph/HDL Subsystem/HDL Algorithm/Mode Selection/State Mode Vector To Index/Subsystem6 ==
  In1 : Inport
  In2 : Inport  Port=2
  In3 : Inport  Port=3
  Bitwise Operator : simulink/Logic and Bit Operations/Bitwise Operator  logicop=XOR  UseBitMask=off  NumInputPorts=2  BitMask=bin2dec('11011001')  BitMaskRealWorld=Stored Integer
  Bitwise Operator1 : simulink/Logic and Bit Operations/Bitwise Operator  logicop=NOR  UseBitMask=off  NumInputPorts=12  BitMask=bin2dec('11011001')  BitMaskRealWorld=Stored Integer
  Demux : Demux  Outputs=12
  Index : Constant  Value=Index  SampleTime=2.5e-07
  Switch : Switch  Criteria=u2 ~= 0
  Out1 : Outport  VectorParamsAs1DForOutWhenUnconnected=off
  wires:
  In1/1 -> Bitwise Operator/1
  In3/1 -> Bitwise Operator/2
  Bitwise Operator/1 -> Demux/1
  Demux/1 -> Bitwise Operator1/1
  Demux/2 -> Bitwise Operator1/2
  Demux/3 -> Bitwise Operator1/3
  Demux/4 -> Bitwise Operator1/4
  Demux/5 -> Bitwise Operator1/5
  Demux/6 -> Bitwise Operator1/6
  Demux/7 -> Bitwise Operator1/7
  Demux/8 -> Bitwise Operator1/8
  Demux/9 -> Bitwise Operator1/9
  Demux/10 -> Bitwise Operator1/10
  Demux/11 -> Bitwise Operator1/11
  Demux/12 -> Bitwise Operator1/12
  In2/1 -> Switch/3
  Bitwise Operator1/1 -> Switch/2
  Switch/1 -> Out1/1
  Index/1 -> Switch/1

== system gmStateSpaceHDL_uz_inverter_3ph/uz_inverter_3ph/HDL Subsystem/HDL Algorithm/Mode Selection/State Mode Vector To Index/Subsystem7 ==
  In1 : Inport
  In2 : Inport  Port=2
  In3 : Inport  Port=3
  Bitwise Operator : simulink/Logic and Bit Operations/Bitwise Operator  logicop=XOR  UseBitMask=off  NumInputPorts=2  BitMask=bin2dec('11011001')  BitMaskRealWorld=Stored Integer
  Bitwise Operator1 : simulink/Logic and Bit Operations/Bitwise Operator  logicop=NOR  UseBitMask=off  NumInputPorts=12  BitMask=bin2dec('11011001')  BitMaskRealWorld=Stored Integer
  Demux : Demux  Outputs=12
  Index : Constant  Value=Index  SampleTime=2.5e-07
  Switch : Switch  Criteria=u2 ~= 0
  Out1 : Outport  VectorParamsAs1DForOutWhenUnconnected=off
  wires:
  In1/1 -> Bitwise Operator/1
  In3/1 -> Bitwise Operator/2
  Bitwise Operator/1 -> Demux/1
  Demux/1 -> Bitwise Operator1/1
  Demux/2 -> Bitwise Operator1/2
  Demux/3 -> Bitwise Operator1/3
  Demux/4 -> Bitwise Operator1/4
  Demux/5 -> Bitwise Operator1/5
  Demux/6 -> Bitwise Operator1/6
  Demux/7 -> Bitwise Operator1/7
  Demux/8 -> Bitwise Operator1/8
  Demux/9 -> Bitwise Operator1/9
  Demux/10 -> Bitwise Operator1/10
  Demux/11 -> Bitwise Operator1/11
  Demux/12 -> Bitwise Operator1/12
  In2/1 -> Switch/3
  Bitwise Operator1/1 -> Switch/2
  Switch/1 -> Out1/1
  Index/1 -> Switch/1

== system gmStateSpaceHDL_uz_inverter_3ph/uz_inverter_3ph/HDL Subsystem/HDL Algorithm/Mode Selection/State Mode Vector To Index/Subsystem8 ==
  In1 : Inport
  In2 : Inport  Port=2
  In3 : Inport  Port=3
  Bitwise Operator : simulink/Logic and Bit Operations/Bitwise Operator  logicop=XOR  UseBitMask=off  NumInputPorts=2  BitMask=bin2dec('11011001')  BitMaskRealWorld=Stored Integer
  Bitwise Operator1 : simulink/Logic and Bit Operations/Bitwise Operator  logicop=NOR  UseBitMask=off  NumInputPorts=12  BitMask=bin2dec('11011001')  BitMaskRealWorld=Stored Integer
  Demux : Demux  Outputs=12
  Index : Constant  Value=Index  SampleTime=2.5e-07
  Switch : Switch  Criteria=u2 ~= 0
  Out1 : Outport  VectorParamsAs1DForOutWhenUnconnected=off
  wires:
  In1/1 -> Bitwise Operator/1
  In3/1 -> Bitwise Operator/2
  Bitwise Operator/1 -> Demux/1
  Demux/1 -> Bitwise Operator1/1
  Demux/2 -> Bitwise Operator1/2
  Demux/3 -> Bitwise Operator1/3
  Demux/4 -> Bitwise Operator1/4
  Demux/5 -> Bitwise Operator1/5
  Demux/6 -> Bitwise Operator1/6
  Demux/7 -> Bitwise Operator1/7
  Demux/8 -> Bitwise Operator1/8
  Demux/9 -> Bitwise Operator1/9
  Demux/10 -> Bitwise Operator1/10
  Demux/11 -> Bitwise Operator1/11
  Demux/12 -> Bitwise Operator1/12
  In2/1 -> Switch/3
  Bitwise Operator1/1 -> Switch/2
  Switch/1 -> Out1/1
  Index/1 -> Switch/1

== matlab function gmStateSpaceHDL_uz_inverter_3ph/uz_inverter_3ph/HDL Subsystem/HDL Algorithm/Mode Selection/Generate Mode Vector ==
  data: x input; u input; modes output; t input
function modes = compute_modes(x,u,t)

  tmp1 = (x(1) + ((-1.0) .* u(1)));
  tmp2 = (((-1.0) .* x(2)) + ((-1.0) .* u(1)));
  tmp3 = (((-1.0) .* x(3)) + ((-1.0) .* u(1)));
  tmp4 = (x(2) + ((-1.0) .* u(1)));
  tmp5 = (((-1.0) .* x(1)) + ((-1.0) .* u(1)));
  tmp6 = (x(3) + ((-1.0) .* u(1)));

  mode1 = (tmp1 > ((0.8) .* (1.0)));
  mode2 = (u(2) > (0.5));
  mode3 = (tmp2 > ((0.8) .* (1.0)));
  mode4 = (u(3) > (0.5));
  mode5 = (tmp3 > ((0.8) .* (1.0)));
  mode6 = (u(4) > (0.5));
  mode7 = (tmp4 > ((0.8) .* (1.0)));
  mode8 = (u(5) > (0.05));
  mode9 = (tmp5 > ((0.8) .* (1.0)));
  mode10 = (u(6) > (0.5));
  mode11 = (tmp6 > ((0.8) .* (1.0)));
  mode12 = (u(7) > (0.05));

  modes = [mode1 mode2 mode3 mode4 mode5 mode6 mode7 mode8 mode9 mode10 mode11 mode12];

end
